simulink model "radio_enlace_conersao_direta"  (R2017a)
settings: Solver=ode45  StartTime=0.0  StopTime=Inf  RelTol=1e-3  EnableMultiTasking=on
libraries: dsparch4 x4, commfilt2 x3, dspstat3 x2, commrflib2 x2, commdigbbndpm3 x2, commsink2 x1, simulink x1, commrandsrc2 x1
settings Model: Creator=ampl  LastModifiedBy=Rubem Pacelli
settings DataIOCC: LimitDataPoints=on  SaveFormat=Array
settings OptimizationCC: LifeSpan=inf
settings DebuggingCC: UnderspecifiedInitializationDetection=Classic  MergeDetectMultiDrivingBlocksExec=none  SolverPrmCheckMsg=warning  SFUnexpectedBacktrackingDiag=warning  SFNoUnconditionalDefaultTransitionDiag=warning  SFExecutionAtInitializationDiag=none
settings HardwareCC: ProdBitPerPointer=32  ProdBitPerSizeT=32  ProdBitPerPtrDiffT=32  ProdLargestAtomicFloat=None  ProdIntDivRoundTo=Undefined  ProdEndianess=Unspecified  ProdWordSize=32  ProdHWDeviceType=32-bit Generic
settings ModelReferenceCC: PropagateSignalLabelsOutOfModel=off
settings GRTTargetCC: TargetLangStandard=C89/C90 (ANSI)  GeneratePreprocessorConditionals=Disable all
settings ConfigComp: CovMetricSettings=dw  CovHtmlReporting=on  CovSaveCumulativeToWorkspaceVar=on  CovSaveSingleToWorkspaceVar=on  CovExternalEMLEnable=off

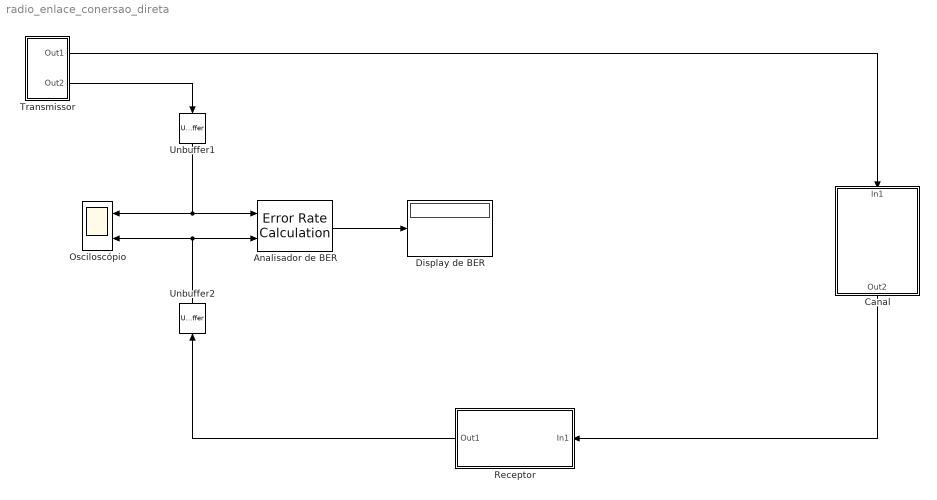
== system radio_enlace_conersao_direta ==
  Analisador de BER : commsink2/Error Rate Calculation  N=24  st_delay=1e3  cp_mode=Entire frame  subframe=[]  PMode=Port  WsName=ErrorVec  RsMode2=off  stop=off  numErr=100  maxBits=1e6
  Canal : Subsystem
  Display de BER : Display
      settings: Format=short_e
  Osciloscópio : Scope  NumInputPorts=2
  Receptor : Subsystem
  Transmissor : Subsystem
  Unbuffer1 : Unbuffer
  Unbuffer2 : Unbuffer
  wires:
  Analisador de BER/1 -> Display de BER/1
  Unbuffer1/1 -> Analisador de BER/1, Osciloscópio/1
  Transmissor/2(Out2) -> Unbuffer1/1
  Transmissor/1(Out1) -> Canal/1(In1)
  Canal/1(Out2) -> Receptor/1(In1)
  Receptor/1(Out1) -> Unbuffer2/1
  Unbuffer2/1 -> Osciloscópio/2, Analisador de BER/2

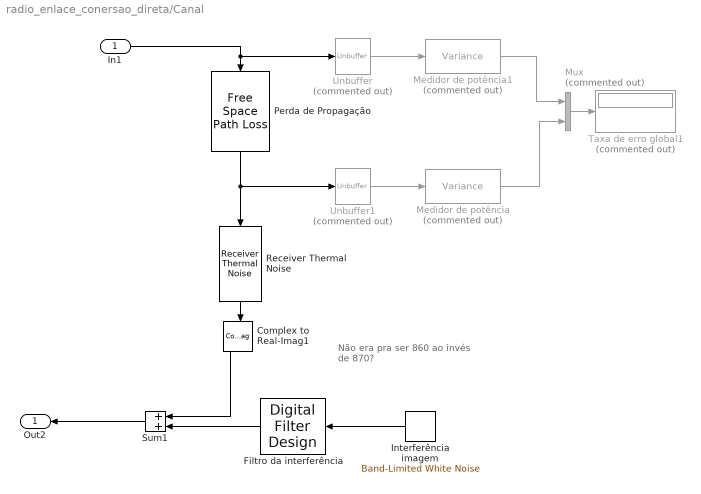
== system radio_enlace_conersao_direta/Canal ==
  note: Não era pra ser 860
      | ao invés de 870?
  In1 : Inport
  Complex to Real-Imag1 : ComplexToRealImag
  Filtro da interferência : dsparch4/Digital Filter Design  mwdsp_browser_bugfix_var=off
  Interferência imagem : simulink/Sources/Band-Limited White Noise  Cov=[0.0001]  Ts=1/4000e6  seed=[23341]
  Medidor de potência : dspstat3/Variance  Commented=on  run=on  reset_popup=None  InputProcessing=Columns as channels (frame based)  directionMode=Each column  dimension=1  roiEnable=off  roiType=Rectangles  roiPortion=Entire ROI  roiOutput=Individual statistics for each ROI  roiFlag=off  roundingMode=Floor  overflowMode=off
      settings: SourceProductName=DSP System Toolbox
  Medidor de potência1 : dspstat3/Variance  Commented=on  run=on  reset_popup=None  InputProcessing=Columns as channels (frame based)  directionMode=Each column  dimension=1  roiEnable=off  roiType=Rectangles  roiPortion=Entire ROI  roiOutput=Individual statistics for each ROI  roiFlag=off  roundingMode=Floor  overflowMode=off
      settings: SourceProductName=DSP System Toolbox
  Mux : Mux  Commented=on  Inputs=2
  Perda de Propagação : commrflib2/Free Space Path Loss  mode=Distance and Frequency  dB=0  d=10  fc=1000
      settings: SourceProductName=Communications System Toolbox  SourceProductBaseCode=CM
  Receiver Thermal Noise : commrflib2/Receiver Thermal Noise  method=Noise figure  ntemp=1000000  nfigure=3  nfactor=2  add290KAntennaNoise=off  seed=67987
      settings: SourceProductName=Communications System Toolbox  SourceProductBaseCode=CM
  Sum1 : Sum  Inputs=+|+
  Taxa de erro global1 : Display  Commented=on
      settings: Format=short_e
  Unbuffer : Unbuffer  Commented=on
  Unbuffer1 : Unbuffer  Commented=on
  Out2 : Outport
  wires:
  Interferência imagem/1 -> Filtro da interferência/1
  Receiver Thermal Noise/1 -> Complex to Real-Imag1/1
  Complex to Real-Imag1/1 -> Sum1/1
  Filtro da interferência/1 -> Sum1/2
  Perda de Propagação/1 -> Unbuffer1/1, Receiver Thermal Noise/1
  Sum1/1 -> Out2/1
  Medidor de potência1/1 -> Mux/1
  In1/1 -> Unbuffer/1, Perda de Propagação/1
  Mux/1 -> Taxa de erro global1/1
  Medidor de potência/1 -> Mux/2
  Unbuffer/1 -> Medidor de potência1/1
  Unbuffer1/1 -> Medidor de potência/1

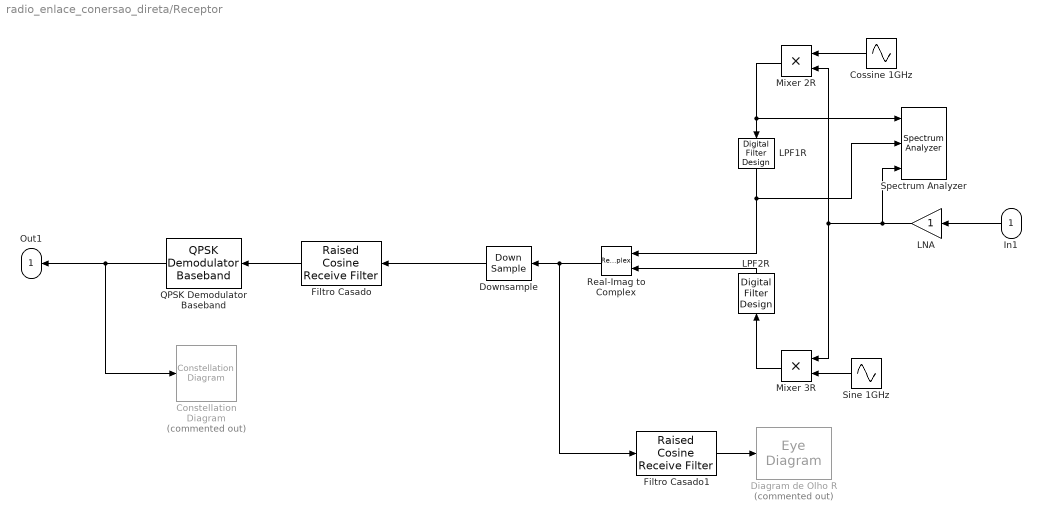
== system radio_enlace_conersao_direta/Receptor ==
  In1 : Inport
  Constellation Diagram : ConstellationDiagram  Commented=on
  Cossine 1GHz : Sin  Frequency=2*pi*(1e9)  Phase=pi/2  Samples=4  SampleTime=1/4000e6
  Diagram de Olho R : EyeDiagram  Tag=EyeDiagram  Commented=on
  Downsample : DownSample  N=10  RateOptions=Allow multirate processing
  Filtro Casado : commfilt2/Raised Cosine Receive Filter  filtType=Square root  R=0.5  filtSpan=10  N=80  downFactor=80  downOffset=18  filterGain=4  InputProcessing=Columns as channels (frame based)  RateOptions=Allow multirate processing  framing=Mute  checkCoeff=off  variableName=rcRxFilt  currentFiltSpan=10  D=5  inputOffset=0  sampMode=Mute  saveAsFlag=0  rateMode=Downsampling  checkGain=Normalized  launchFVT=on  roundingMode=Floor  overflowMode=off  coeffDataTypeStr=Inherit: Same word length as input  coeffMin=[]  coeffMax=[]  coeffLastDataTypeStr=Inherit: Same word length as input  accumDataTypeStr=Inherit: Same as product output  accumLastDataTypeStr=Inherit: Same as product output  outputDataTypeStr=Inherit: Same as accumulator  outputMin=[]  outputMax=[]  outputLastDataTypeStr=Inherit: Same as accumulator
  Filtro Casado1 : commfilt2/Raised Cosine Receive Filter  filtType=Square root  R=0.5  filtSpan=10  N=800  downFactor=10  downOffset=0  filterGain=4  InputProcessing=Columns as channels (frame based)  RateOptions=Allow multirate processing  framing=Mute  checkCoeff=off  variableName=rcRxFilt1  currentFiltSpan=10  D=5  inputOffset=0  sampMode=Mute  saveAsFlag=0  rateMode=Downsampling  checkGain=Normalized  launchFVT=on  roundingMode=Floor  overflowMode=off  coeffDataTypeStr=Inherit: Same word length as input  coeffMin=[]  coeffMax=[]  coeffLastDataTypeStr=Inherit: Same word length as input  accumDataTypeStr=Inherit: Same as product output  accumLastDataTypeStr=Inherit: Same as product output  outputDataTypeStr=Inherit: Same as accumulator  outputMin=[]  outputMax=[]  outputLastDataTypeStr=Inherit: Same as accumulator
  LNA : Gain
  LPF1R : dsparch4/Digital Filter Design  mwdsp_browser_bugfix_var=off
  LPF2R : dsparch4/Digital Filter Design  mwdsp_browser_bugfix_var=off
  Mixer 2R : Product  RndMeth=Zero
  Mixer 3R : Product  RndMeth=Zero
  QPSK Demodulator Baseband : commdigbbndpm3/QPSK Demodulator Baseband  OutType=Bit  DecType=Hard decision  VarSource=Dialog  Variance=1  Dec=Gray  Ph=pi/4  outDtype1=Inherit via internal rule  outDtype2=Inherit via internal rule  derotateFactorWordLen=16  derotateFactorDataTypeStr=Inherit: Same word length as input  derotateFactorLastDataTypeStr=Inherit: Same word length as input
  Real-Imag to Complex : RealImagToComplex
  Sine 1GHz : Sin  Frequency=2*pi*(1e9)  Phase=pi  Samples=4  SampleTime=1/4000e6
  Spectrum Analyzer : SpectrumAnalyzer  NumInputPorts=3
  Out1 : Outport
  wires:
  In1/1 -> LNA/1
  Cossine 1GHz/1 -> Mixer 2R/1
  Mixer 2R/1 -> LPF1R/1, Spectrum Analyzer/1
  Filtro Casado/1 -> QPSK Demodulator Baseband/1
  LNA/1 -> Spectrum Analyzer/3, Mixer 3R/1, Mixer 2R/2
  QPSK Demodulator Baseband/1 -> Constellation Diagram/1, Out1/1
  LPF2R/1 -> Real-Imag to Complex/2
  LPF1R/1 -> Spectrum Analyzer/2, Real-Imag to Complex/1
  Mixer 3R/1 -> LPF2R/1
  Sine 1GHz/1 -> Mixer 3R/2
  Real-Imag to Complex/1 -> Filtro Casado1/1, Downsample/1
  Downsample/1 -> Filtro Casado/1
  Filtro Casado1/1 -> Diagram de Olho R/1

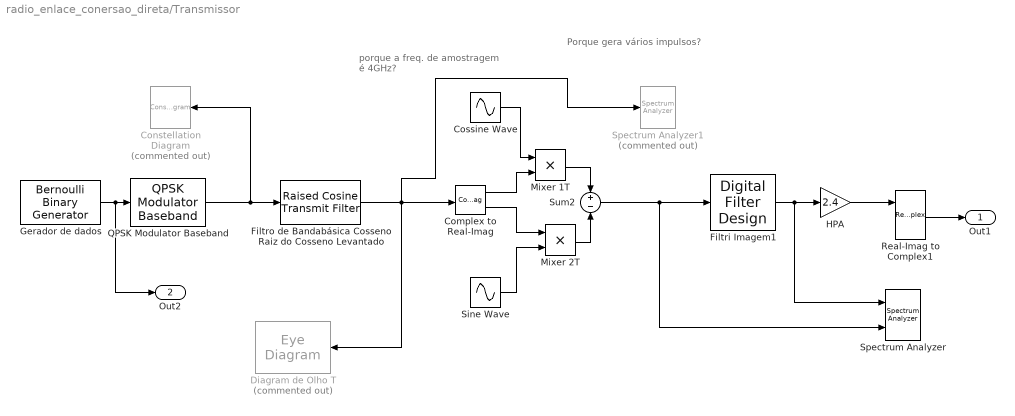
== system radio_enlace_conersao_direta/Transmissor ==
  note: porque a freq. de amostragem é 4GHz?
  note: Porque gera vários impulsos?
  Complex to Real-Imag : ComplexToRealImag
  Constellation Diagram : ConstellationDiagram  Commented=on
  "Cossine Wave " : Sin  Frequency=2*pi*(1000e6)  Phase=pi/2  Samples=4  SampleTime=1/4000e6
  Diagram de Olho T : EyeDiagram  Tag=EyeDiagram  Commented=on
  Filtri Imagem1 : dsparch4/Digital Filter Design  mwdsp_browser_bugfix_var=off
  Filtro de Bandabásica Cosseno Raiz do Cosseno Levantado : commfilt2/Raised Cosine Transmit Filter  filtType=Square root  R=0.5  filtSpan=10  N=80  filterGain=1  InputProcessing=Columns as channels (frame based)  RateOptions=Allow multirate processing  framing=Mute  checkCoeff=off  variableName=rcTxFilt  checkGain=Normalized  sampMode=Mute  saveAsFlag=0  currentFiltSpan=10  D=5  launchFVT=on  roundingMode=Floor  overflowMode=off  coeffDataTypeStr=Inherit: Same word length as input  coeffMin=[]  coeffMax=[]  coeffLastDataTypeStr=Inherit: Same word length as input  outputDataTypeStr=Inherit: Same as accumulator  outputMin=[]  outputMax=[]  outputLastDataTypeStr=Inherit: Same as accumulator
  Gerador de dados : commrandsrc2/Bernoulli Binary Generator  P=0.5  seed=61  Ts=1/10e6  frameBased=on  sampPerFrame=2  orient=off  outDataType=double
  HPA : Gain  Gain=2.4
  Mixer 1T : Product  RndMeth=Zero
  Mixer 2T : Product  RndMeth=Zero
  QPSK Modulator Baseband : commdigbbndpm3/QPSK Modulator Baseband  InType=Bit  Enc=Gray  Ph=pi/4  outDtype=double  outWordLen=16  outUDDataType=sfix(16)  outFracLenMode=Best precision  outFracLen=15  outDataTypeStr=double  outLastDataTypeStr=double
  Real-Imag to Complex1 : RealImagToComplex
  Sine Wave : Sin  Frequency=2*pi*(1000e6)  Samples=4  SampleTime=1/4000e6
  Spectrum Analyzer : SpectrumAnalyzer  NumInputPorts=2
  Spectrum Analyzer1 : SpectrumAnalyzer  Commented=on
  Sum2 : Sum  Inputs=+|-
  Out1 : Outport
  Out2 : Outport  Port=2
  wires:
  Mixer 2T/1 -> Sum2/2
  Mixer 1T/1 -> Sum2/1
  Complex to Real-Imag/2 -> Mixer 2T/1
  Sine Wave/1 -> Mixer 2T/2
  Filtro de Bandabásica Cosseno Raiz do Cosseno Levantado/1 -> Spectrum Analyzer1/1, Diagram de Olho T/1, Complex to Real-Imag/1
  Gerador de dados/1 -> Out2/1, QPSK Modulator Baseband/1
  Complex to Real-Imag/1 -> Mixer 1T/2
  "Cossine Wave "/1 -> Mixer 1T/1
  Real-Imag to Complex1/1 -> Out1/1
  Sum2/1 -> Spectrum Analyzer/2, Filtri Imagem1/1
  Filtri Imagem1/1 -> Spectrum Analyzer/1, HPA/1
  HPA/1 -> Real-Imag to Complex1/1
  QPSK Modulator Baseband/1 -> Constellation Diagram/1, Filtro de Bandabásica Cosseno Raiz do Cosseno Levantado/1
